simulink model "PIDcontroller_model"  (R2017a)
settings: Solver=VariableStepAuto  StartTime=0.0  StopTime=simulatietijd  MaxStep=1e-3  RelTol=1e-3  EnableMultiTasking=on
values from neighbouring files (symbols this model uses):
  K_2 = 3    [PIDcontroller.m]
  K_m = 1    [PIDcontroller.m]
  Kc = Kc_help(i)    [PIDTuning.m]    (also in PIDcontroller.m = 5; controlWithMeasurementDelay.m = 2)
  t_step = 5    [PIDcontroller.m]    (also in controlWithMeasurementDelay.m = 1800)
  tau1 = 2    [PIDTuning.m]    (also in PIDcontroller.m; margin.m)
  tau2 = 6    [PIDTuning.m]    (also in PIDcontroller.m; margin.m)
  tau_d = tau_d_help(i)    [PIDcontroller.m]
  tau_i = 1/3*Kc    (= 1.66666666667)    [PIDcontroller.m]
  tau_m = 0.2    [PIDcontroller.m]
  y_sp_na = 1    [PIDcontroller.m]
  y_sp_voor = 0    [PIDcontroller.m]
libraries: simulink x1
settings Model: Creator=wrquaghe  LastModifiedBy=geert
settings DataIOCC: LimitDataPoints=on
settings OptimizationCC: LifeSpan=inf
settings DebuggingCC: AllowSymbolicDim=off  SFUnexpectedBacktrackingDiag=warning  SFNoUnconditionalDefaultTransitionDiag=warning  SFExecutionAtInitializationDiag=none
settings ModelReferenceCC: PropagateSignalLabelsOutOfModel=off
settings GRTTargetCC: TargetLangStandard=C89/C90 (ANSI)
settings ConfigComp: CovMetricSettings=dw  CovHtmlReporting=on  CovSaveCumulativeToWorkspaceVar=on  CovSaveSingleToWorkspaceVar=on  CovExternalEMLEnable=off

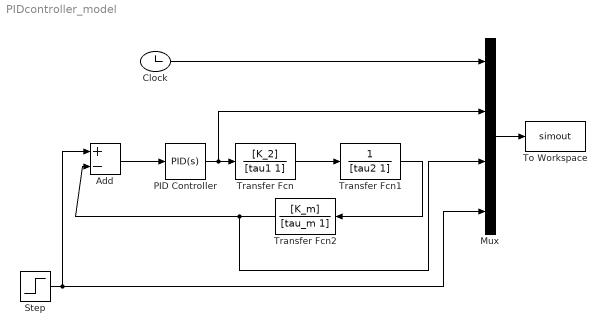
== system PIDcontroller_model ==
  Add : Sum  Inputs=+-
  Clock : Clock
  Mux : Mux
  PID Controller : simulink/Continuous/PID Controller  Controller=PID  TimeDomain=Continuous-time  SampleTime=-1  IntegratorMethod=Forward Euler  FilterMethod=Forward Euler  Form=Parallel  UseFilter=on  ControllerParametersSource=internal  P=Kc  I=tau_i  D=tau_d  N=100  InitialConditionSource=internal  InitialConditionForIntegrator=0  InitialConditionForFilter=0  ExternalReset=none  LimitOutput=off  UpperSaturationLimit=inf  LowerSaturationLimit=-inf  LinearizeAsGain=on  AntiWindupMode=none  Kb=1  TrackingMode=off  Kt=1  PParamMin=[]  PParamMax=[]  IParamMin=[]  IParamMax=[]  DParamMin=[]  DParamMax=[]  NParamMin=[]  NParamMax=[]  KbParamMin=[]  KbParamMax=[]  KtParamMin=[]  KtParamMax=[]  POutMin=[]  POutMax=[]  IOutMin=[]  IOutMax=[]  DOutMin=[]  DOutMax=[]  NOutMin=[]  NOutMax=[]  KbOutMin=[]  KbOutMax=[]  KtOutMin=[]  KtOutMax=[]  IntegratorOutMin=[]  IntegratorOutMax=[]  FilterOutMin=[]  FilterOutMax=[]  SumOutMin=[]  SumOutMax=[]  SumI1OutMin=[]  SumI1OutMax=[]  SumI2OutMin=[]  SumI2OutMax=[]  SumI3OutMin=[]  SumI3OutMax=[]  SumDOutMin=[]  SumDOutMax=[]  SaturationOutMin=[]  SaturationOutMax=[]  IntegratorContinuousStateAttributes=''  IntegratorStateMustResolveToSignalObject=off  IntegratorRTWStateStorageClass=Auto  FilterContinuousStateAttributes=''  FilterStateMustResolveToSignalObject=off  FilterRTWStateStorageClass=Auto  DifferentiatorICPrevScaledInput=0  DifferentiatorOutMin=[]  DifferentiatorOutMax=[]  InitialConditionSetting=State (most efficient)
  Step : Step  Time=t_step  Before=y_sp_voor  After=y_sp_na  SampleTime=0
  To Workspace : ToWorkspace  VariableName=simout  SampleTime=-1
  Transfer Fcn : TransferFcn  Numerator=[K_2]  Denominator=[tau1 1]
  Transfer Fcn1 : TransferFcn  Denominator=[tau2 1]
  Transfer Fcn2 : TransferFcn  Numerator=[K_m]  Denominator=[tau_m 1]
  wires:
  Clock/1 -> Mux/1
  Step/1 -> Add/1, Mux/4
  Add/1 -> PID Controller/1
  PID Controller/1 -> Mux/2, Transfer Fcn/1
  Mux/1 -> To Workspace/1
  Transfer Fcn/1 -> Transfer Fcn1/1
  Transfer Fcn1/1 -> Transfer Fcn2/1
  Transfer Fcn2/1 -> Mux/3, Add/2
